simulink model "imagedetector"  (R2021a)
settings: Solver=VariableStepAuto  StartTime=0.0  StopTime=10.0  RelTol=1e-3
model workspace (MAT data in the model file):
  SL_ROS_VariableLengthArrays_MaxSizes.CommonInfo.ArrayTruncateAction = 'EmitWarning'
  SL_ROS_VariableLengthArrays_MaxSizes.MsgTypeMap = containers.Map
  SL_ROS_VariableLengthArrays_MaxSizes.MsgTypeMap.serialization.keys = {'sensor_msgs/Image'}
  SL_ROS_VariableLengthArrays_MaxSizes.MsgTypeMap.serialization.values{1}(1).PropertyName = 'Data'
  SL_ROS_VariableLengthArrays_MaxSizes.MsgTypeMap.serialization.values{1}(1).DataType = 'uint8'
  SL_ROS_VariableLengthArrays_MaxSizes.MsgTypeMap.serialization.values{1}(1).MaxLength = 921600
  SL_ROS_VariableLengthArrays_MaxSizes.MsgTypeMap.serialization.values{1}(2).PropertyName = 'Encoding'
  SL_ROS_VariableLengthArrays_MaxSizes.MsgTypeMap.serialization.values{1}(2).DataType = 'uint8'
  SL_ROS_VariableLengthArrays_MaxSizes.MsgTypeMap.serialization.values{1}(2).MaxLength = 128
  SL_ROS_VariableLengthArrays_MaxSizes.MsgTypeMap.serialization.uniformity = 0
  SL_ROS_VariableLengthArrays_MaxSizes.MsgTypeMap.serialization.keyType = 'char'
  SL_ROS_VariableLengthArrays_MaxSizes.MsgTypeMap.serialization.valueType = 'any'
undefined symbols (not defined in the file or in its folder): ModelName, ModelName_SL_Info, Pose
libraries: robotlib x4
settings Model: Creator=lambdavary  LastModifiedBy=lambdavary

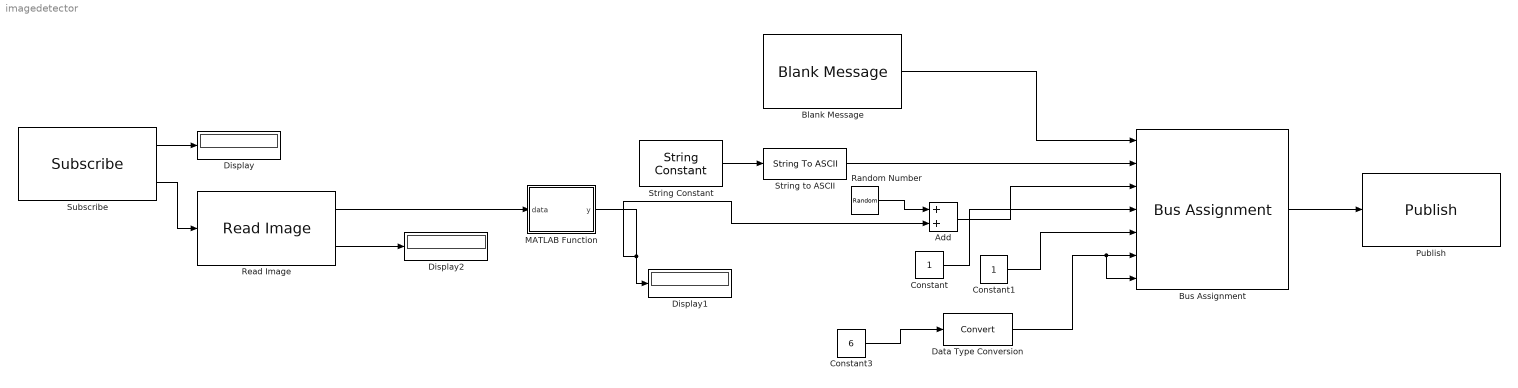
== system imagedetector ==
  Add : Sum
  Blank Message : robotlib/Blank Message  messageClass=Message  entityType=gazebo_msgs/ModelState  messageType=gazebo_msgs/ModelState  SampleTime=inf  legacyBusStruct=off
  Bus Assignment : BusAssignment  AssignedSignals=ModelName,Pose.Position.X,Pose.Position.Y,Pose.Position.Z,ModelName_SL_Info.CurrentLength,ModelName_SL_Info.ReceivedLength
  Constant : Constant
  Constant1 : Constant
  Constant3 : Constant  Value=6
  Data Type Conversion : DataTypeConversion
  Display : Display
  Display1 : Display
  Display2 : Display
  MATLAB Function : MATLAB Function  TreatAsAtomicUnit=on
  Publish : robotlib/Publish  topicSource=Select from ROS network  topic=/gazebo/set_model_state  messageType=gazebo_msgs/ModelState  legacyBusStruct=off  messageQueueLength=1
  Random Number : RandomNumber  Variance=0.5  SampleTime=0.1
  Read Image : robotlib/Read Image  MaximumImageSize=[480, 640]  ImageEncoding=rgb8  ShowAlphaOutput=off  ShowErrorCodeOutput=on  VariableSizeOutputs=off
      settings: SourceProductBaseCode=RR
  String Constant : StringConstant  String="\"tanker\""
  String to ASCII : StringToASCII  OutputVectorSize=128
  Subscribe : robotlib/Subscribe  topicSource=Select from ROS network  topic=/camera/image_raw  messageType=sensor_msgs/Image  SampleTime=-1  legacyBusStruct=off  messageQueueLength=1
  wires:
  Subscribe/1 -> Display/1
  Subscribe/2 -> Read Image/1
  Read Image/2 -> Display2/1
  Read Image/1 -> MATLAB Function/1(data)
  Data Type Conversion/1 -> Bus Assignment/7, Bus Assignment/6
  Random Number/1 -> Add/1
  String to ASCII/1 -> Bus Assignment/2
  Add/1 -> Bus Assignment/3
  Constant3/1 -> Data Type Conversion/1
  String Constant/1 -> String to ASCII/1
  Blank Message/1 -> Bus Assignment/1
  Bus Assignment/1 -> Publish/1
  MATLAB Function/1(y) -> Display1/1, Add/2
  Constant/1 -> Bus Assignment/4
  Constant1/1 -> Bus Assignment/5

== matlab function imagedetector/MATLAB Function ==
  data: y output; data input
function y = fcn(data)
[centersDark,radiiDark] = imfindcircles(data,[10 300],'ObjectPolarity','dark', 'Sensitivity',0.92);
xPos = 0
if ~isempty(centersDark)
xPos = -5.983*10^-7*radiiDark(1)^5 + 0.0001086*radiiDark(1)^4 - 0.00788*radiiDark(1)^3 + 0.292*radiiDark(1)^2 - 5.812*radiiDark(1) + 59;
yPos = (320-centersDark(1))/(2*radiiDark(1));
zPos = (240-centersDark(2))/(1.5*radiiDark(1));
end
y = xPos;
